simulink model "LongitudinalTFs"  (R2020a)
settings: Solver=VariableStepAuto  StartTime=0.0  StopTime=500  RelTol=1e-3
settings Model: Creator=OZAN  LastModifiedBy=OZAN

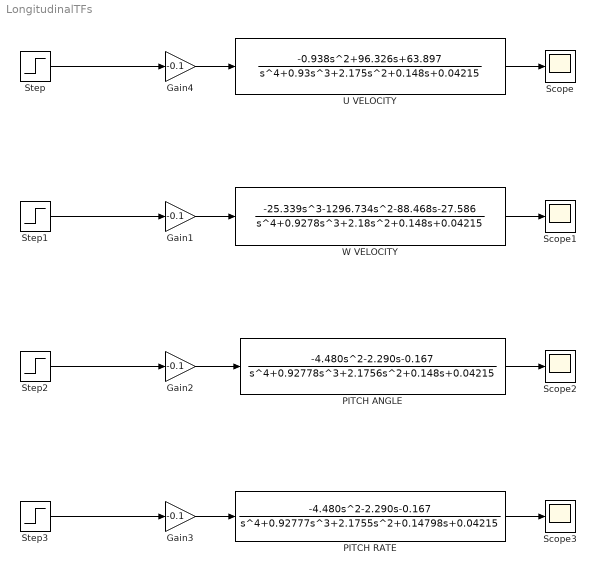
== system LongitudinalTFs ==
  Gain{1..4} (4 alike) : Gain  Gain=-0.1
  PITCH ANGLE : TransferFcn  Numerator=[-4.480,-2.290,-0.167]  Denominator=[1,0.92778,2.1756,0.148,0.04215]
  PITCH RATE : TransferFcn  Numerator=[0,0,-4.480,-2.290,-0.167]  Denominator=[1,0.92777,2.1755,0.14798,0.04215]
  Scope{,1..3} (4 alike) : Scope
  Step{,1..3} (4 alike) : Step  SampleTime=0
  U VELOCITY : TransferFcn  Numerator=[-0.938,96.326,63.897]  Denominator=[1,0.93,2.175,0.148,0.04215]
  W VELOCITY : TransferFcn  Numerator=[-25.339,-1296.734,-88.468,-27.586]  Denominator=[1,0.9278,2.18,0.148,0.04215]
  wires:
  U VELOCITY/1 -> Scope/1
  PITCH RATE/1 -> Scope3/1
  PITCH ANGLE/1 -> Scope2/1
  W VELOCITY/1 -> Scope1/1
  Gain4/1 -> U VELOCITY/1
  Gain1/1 -> W VELOCITY/1
  Gain2/1 -> PITCH ANGLE/1
  Gain3/1 -> PITCH RATE/1
  Step/1 -> Gain4/1
  Step1/1 -> Gain1/1
  Step2/1 -> Gain2/1
  Step3/1 -> Gain3/1
